simulink subsystem "Encoders"  (R2024a)
settings: Solver=VariableStepAuto  StartTime=0.0  StopTime=10.0  RelTol=1e-3
undefined symbols (not defined in the file or in its folder): collocated
settings Model: Creator=20201350  LastModifiedBy=20201350

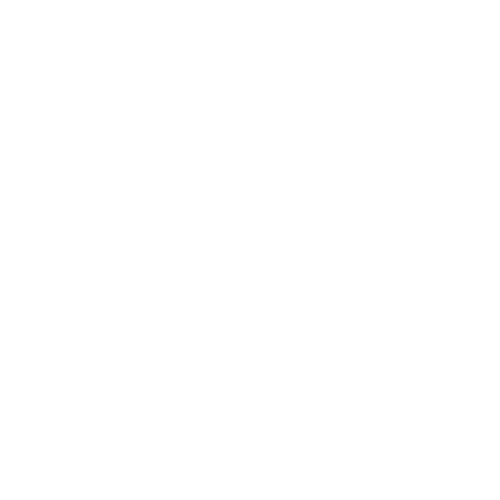
[thumbnail: Simulink's stored preview of the top-level diagram]
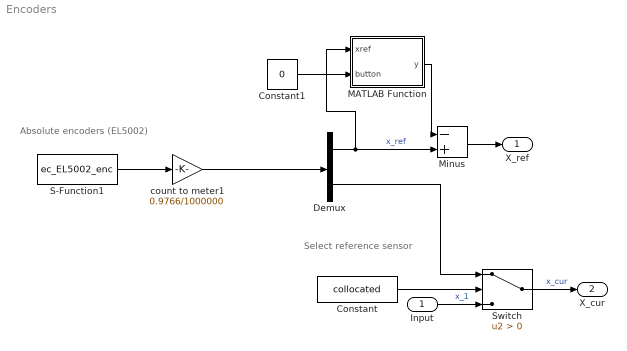
== system Encoders ==
  note: Select reference sensor
  note: Absolute encoders (EL5002)
  Input : Inport
  Constant : Constant  Value=collocated
  Constant1 : Constant  Value=0
  Demux : Demux  Outputs=2
  MATLAB Function : MATLAB Function  TreatAsAtomicUnit=on
  Minus : Sum  Inputs=-+
  S-Function1 : S-Function  FunctionName=ec_EL5002_enc  Parameters=ENC_LINK_ID  SFunctionDeploymentMode=off  EnableBusSupport=off
  Switch : Switch  Criteria=u2 > Threshold  SaturateOnIntegerOverflow=off  InputSameDT=off
  count to meter1 : Gain  Gain=0.9766/1000000
  X_ref : Outport
  X_cur : Outport  Port=2
  wires:
  S-Function1/1 -> count to meter1/1
  count to meter1/1 -> Demux/1
  Demux/2 -> Switch/1
  Switch/1 -> X_cur/1  "x_cur"
  Input/1 -> Switch/3  "x_1"
  Constant/1 -> Switch/2
  Demux/1 -> Minus/2, MATLAB Function/1(xref)  "x_ref"
  Minus/1 -> X_ref/1
  MATLAB Function/1(y) -> Minus/1
  Constant1/1 -> MATLAB Function/2(button)

== matlab function Encoders/MATLAB Function ==
  data: xref input; y output; button input
function y = fcn(xref, button)
if button
    y = xref;
end
